simulink model "ODR_schematic"  (R2019b)
settings: Solver=VariableStepAuto  StartTime=0.0  StopTime=10.0  RelTol=1e-3
settings Model: Creator=Já  LastModifiedBy=Já

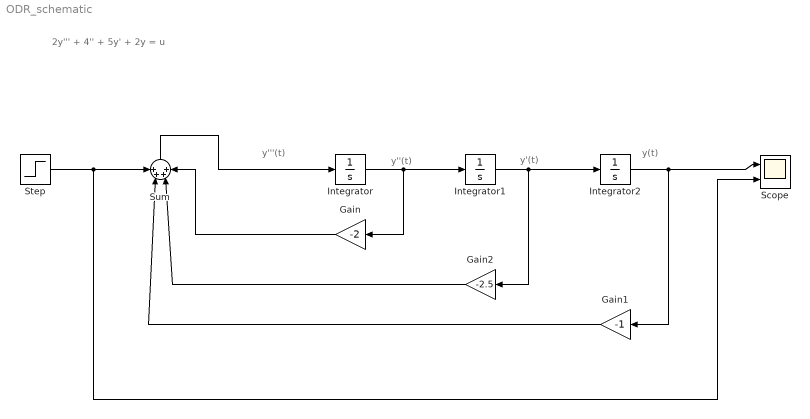
== system ODR_schematic ==
  note: y'''(t)
  note: y''(t)
  note: y'(t)
  note: y(t)
  note: 2y''' + 4'' + 5y' + 2y = u
  Gain : Gain  Gain=-2
  Gain1 : Gain  Gain=-1
  Gain2 : Gain  Gain=-2.5
  Integrator : Integrator
  Integrator1 : Integrator
  Integrator2 : Integrator
  Scope : Scope  NumInputPorts=2
  Step : Step  SampleTime=0
  Sum : Sum  Inputs=++++
  wires:
  Integrator1/1 -> Gain2/1, Integrator2/1
  Integrator/1 -> Gain/1, Integrator1/1
  Integrator2/1 -> Gain1/1, Scope/1
  Sum/1 -> Integrator/1
  Gain/1 -> Sum/4
  Gain2/1 -> Sum/3
  Gain1/1 -> Sum/2
  Step/1 -> Scope/2, Sum/1
